simulink model "mavsim_chap7"  (R2014a)
settings: Solver=ode15s  StartTime=0.0  StopTime=10000  RelTol=1e-3
InitFcn:
  | param_chap6
undefined symbols (not defined in the file): autopilot, drawUAV, forces_moments, gps, P, plotmavstatevariables, sensors, true_states
libraries: simulink x6
settings Model: Creator=beard  LastModifiedBy=danst_000
settings DataIOCC: SignalLoggingSaveFormat=ModelDataLogs
settings OptimizationCC: ExpressionDepthLimit=2147483647  InitFltsAndDblsToZero=on
settings DebuggingCC: UnderspecifiedInitializationDetection=Classic  FcnCallInpInsideContextMsg=UseLocalSettings  StateNameClashWarn=warning
settings GRTTargetCC: CombineOutputUpdateFcns=off  GRTInterface=on

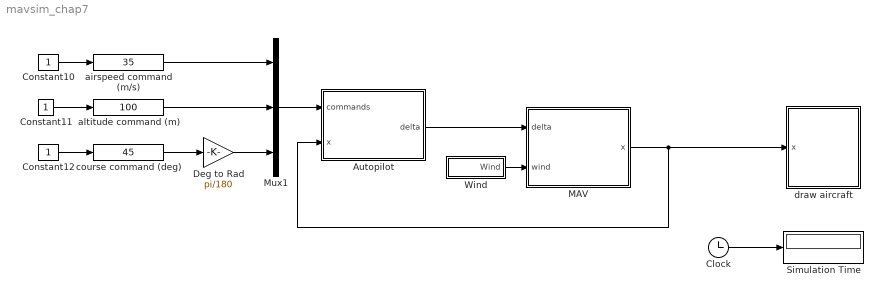
== system mavsim_chap7 ==
  Autopilot : Subsystem
      mask Display: image(imread('kestrel.jpg'))
  Clock : Clock
  Constant10 : Constant
  Constant11 : Constant
  Constant12 : Constant
  Deg to Rad : Gain  Gain=pi/180
  MAV : Subsystem
      mask Display: image(imread('batcam.png'))
  Mux1 : Mux  Inputs=3
  Simulation Time : Display
  Wind : Subsystem
  airspeed command (m/s) : simulink/Math Operations/Slider Gain  low=5  gain=35  high=50
  altitude command (m) : simulink/Math Operations/Slider Gain  low=0  gain=100  high=500
  course command (deg) : simulink/Math Operations/Slider Gain  low=-360  gain=45  high=360
  draw aircraft : Subsystem
      mask Display: image(imread('tv.jpg'))
  wires:
  Clock/1 -> Simulation Time/1
  Wind/1(Wind) -> MAV/2(wind)
  MAV/1(x) -> draw aircraft/1(x), Autopilot/2(x)
  Autopilot/1(delta) -> MAV/1(delta)
  Constant10/1 -> airspeed command (m/s)/1
  Constant11/1 -> altitude command (m)/1
  Constant12/1 -> course command (deg)/1
  course command (deg)/1 -> Deg to Rad/1
  altitude command (m)/1 -> Mux1/2
  airspeed command (m/s)/1 -> Mux1/1
  Mux1/1 -> Autopilot/1(commands)
  Deg to Rad/1 -> Mux1/3

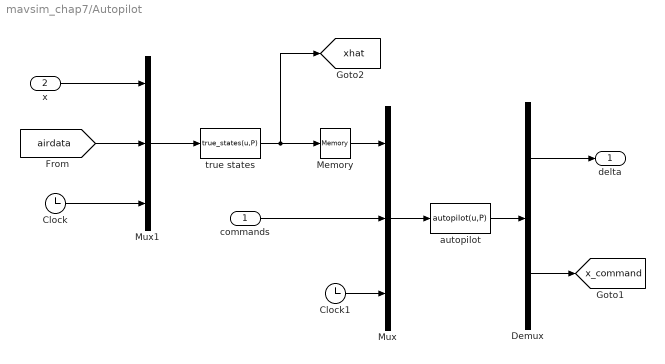
== system mavsim_chap7/Autopilot ==
  commands : Inport
  x : Inport  Port=2
  Clock : Clock
  Clock1 : Clock
  Demux : Demux  Outputs=[4;12]
  Memory : Memory
  Mux : Mux  Inputs=3
  Mux1 : Mux  Inputs=3
  autopilot : MATLABFcn  MATLABFcn=autopilot(u,P)  OutputDimensions=4+12  SampleTime=P.Ts
  true states : MATLABFcn  MATLABFcn=true_states(u,P)  OutputDimensions=19  SampleTime=P.Ts
  delta : Outport
  tag scope: x_command=global, xhat=global
  wires:
  Mux/1 -> autopilot/1
  Clock/1 -> Mux1/3
  autopilot/1 -> Demux/1
  Demux/1 -> delta/1
  Demux/2 -> [x_command]
  commands/1 -> Mux/2
  Mux1/1 -> true states/1
  x/1 -> Mux1/1
  true states/1 -> [xhat], Memory/1
  [airdata] -> Mux1/2
  Memory/1 -> Mux/1
  Clock1/1 -> Mux/3

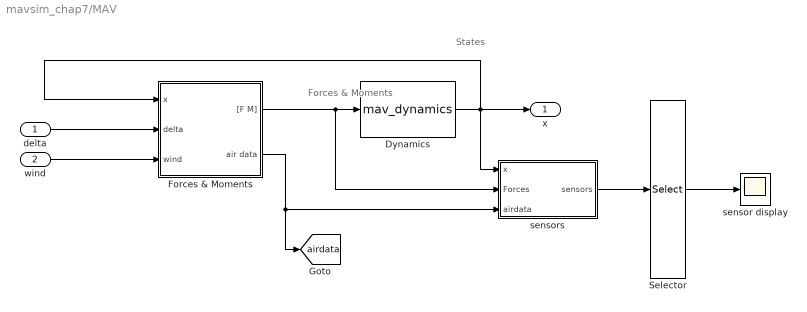
== system mavsim_chap7/MAV ==
  note: Forces & Moments
  note: States
  delta : Inport
  wind : Inport  Port=2
  Dynamics : S-Function  FunctionName=mav_dynamics  Parameters=P  EnableBusSupport=off
  Forces & Moments : Subsystem
  Selector : Selector  InputPortWidth=13  Indices=2
  sensor display : Scope
      settings: TimeRange=45  YMin=-1.5  YMax=3.5
  sensors : Subsystem
  x : Outport
  tag scope: airdata=global
  wires:
  Dynamics/1 -> Forces & Moments/1(x), x/1, sensors/1(x)
  Forces & Moments/1("[F M]") -> Dynamics/1, sensors/2(Forces)
  Forces & Moments/2(air data) -> [airdata], sensors/3(airdata)
  delta/1 -> Forces & Moments/2(delta)
  wind/1 -> Forces & Moments/3(wind)
  sensors/1(sensors) -> Selector/1
  Selector/1 -> sensor display/1

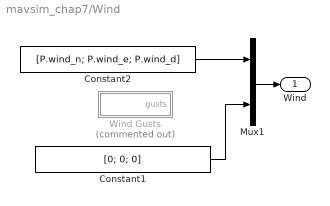
== system mavsim_chap7/Wind ==
  Constant1 : Constant  Value=[0; 0; 0]
  Constant2 : Constant  Value=[P.wind_n; P.wind_e; P.wind_d]
  Mux1 : Mux  Inputs=2
  Wind Gusts : Subsystem  Commented=on
  Wind : Outport
  wires:
  Constant2/1 -> Mux1/1
  Mux1/1 -> Wind/1
  Constant1/1 -> Mux1/2

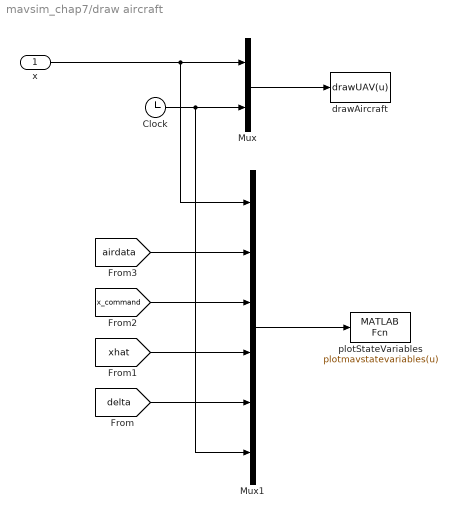
== system mavsim_chap7/draw aircraft ==
  x : Inport
  Clock : Clock
  Mux : Mux  Inputs=2
  Mux1 : Mux  Inputs=6
  drawAircraft : MATLABFcn  MATLABFcn=drawUAV(u)  OutputDimensions=0  SampleTime=0.1
  plotStateVariables : MATLABFcn  MATLABFcn=plotmavstatevariables(u)  OutputDimensions=0  SampleTime=0.1
  wires:
  [airdata] -> Mux1/2
  [delta] -> Mux1/5
  [x_command] -> Mux1/3
  [xhat] -> Mux1/4
  Mux1/1 -> plotStateVariables/1
  Clock/1 -> Mux1/6, Mux/2
  x/1 -> Mux1/1, Mux/1
  Mux/1 -> drawAircraft/1

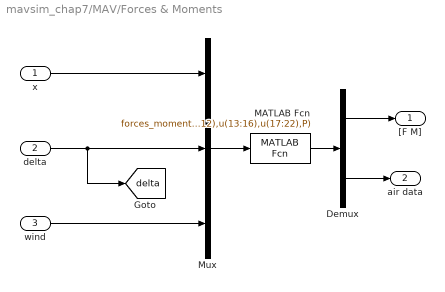
== system mavsim_chap7/MAV/Forces & Moments ==
  x : Inport
  delta : Inport  Port=2
  wind : Inport  Port=3
  Demux : Demux  Outputs=[6;6]
  MATLAB Fcn : MATLABFcn  MATLABFcn=forces_moments(u(1:12),u(13:16),u(17:22),P)  OutputDimensions=12
  Mux : Mux  Inputs=3
  "[F M]" : Outport
  air data : Outport  Port=2
  tag scope: delta=global
  wires:
  x/1 -> Mux/1
  delta/1 -> [delta], Mux/2
  wind/1 -> Mux/3
  MATLAB Fcn/1 -> Demux/1
  Demux/1 -> "[F M]"/1
  Mux/1 -> MATLAB Fcn/1
  Demux/2 -> air data/1

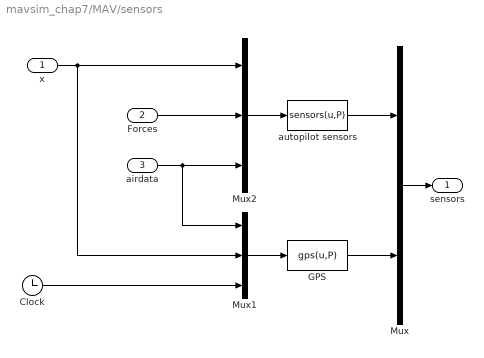
== system mavsim_chap7/MAV/sensors ==
  x : Inport
  Forces : Inport  Port=2
  airdata : Inport  Port=3
  Clock : Clock
  GPS : MATLABFcn  MATLABFcn=gps(u,P)  OutputDimensions=5  SampleTime=P.Ts_gps
  Mux : Mux  Inputs=2
  Mux1 : Mux  Inputs=3
  Mux2 : Mux  Inputs=3
  autopilot sensors : MATLABFcn  MATLABFcn=sensors(u,P)  OutputDimensions=8  SampleTime=P.Ts
  sensors : Outport
  wires:
  autopilot sensors/1 -> Mux/1
  GPS/1 -> Mux/2
  Mux1/1 -> GPS/1
  Clock/1 -> Mux1/3
  Mux2/1 -> autopilot sensors/1
  Forces/1 -> Mux2/2
  airdata/1 -> Mux2/3, Mux1/1
  Mux/1 -> sensors/1
  x/1 -> Mux2/1, Mux1/2

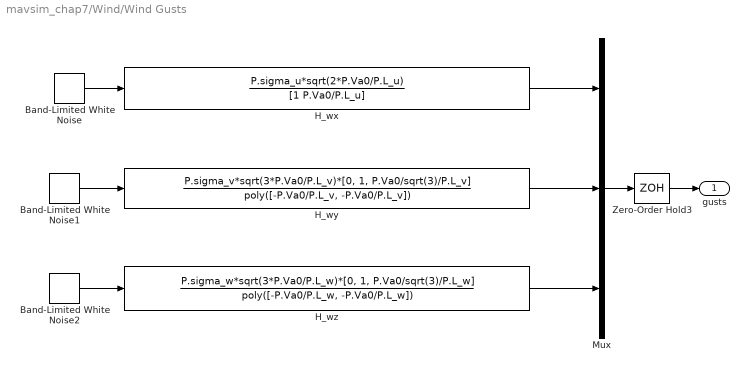
== system mavsim_chap7/Wind/Wind Gusts ==
  Band-Limited White Noise : simulink/Sources/Band-Limited White Noise  Cov=[1]  Ts=P.Ts  seed=[23341]
  Band-Limited White Noise1 : simulink/Sources/Band-Limited White Noise  Cov=[1]  Ts=P.Ts  seed=[23341]
  Band-Limited White Noise2 : simulink/Sources/Band-Limited White Noise  Cov=[1]  Ts=P.Ts  seed=[23341]
  H_wx : TransferFcn  Numerator=P.sigma_u*sqrt(2*P.Va0/P.L_u)  Denominator=[1 P.Va0/P.L_u]
  H_wy : TransferFcn  Numerator=P.sigma_v*sqrt(3*P.Va0/P.L_v)*[0, 1, P.Va0/sqrt(3)/P.L_v]  Denominator=poly([-P.Va0/P.L_v, -P.Va0/P.L_v])
  H_wz : TransferFcn  Numerator=P.sigma_w*sqrt(3*P.Va0/P.L_w)*[0, 1, P.Va0/sqrt(3)/P.L_w]  Denominator=poly([-P.Va0/P.L_w, -P.Va0/P.L_w])
  Mux : Mux  Inputs=3
  Zero-Order Hold3 : ZeroOrderHold  SampleTime=P.Ts
  gusts : Outport
  wires:
  Zero-Order Hold3/1 -> gusts/1
  Mux/1 -> Zero-Order Hold3/1
  Band-Limited White Noise2/1 -> H_wz/1
  H_wz/1 -> Mux/3
  Band-Limited White Noise1/1 -> H_wy/1
  H_wy/1 -> Mux/2
  Band-Limited White Noise/1 -> H_wx/1
  H_wx/1 -> Mux/1
